simulink model "lookup_nD_TestGen18"  (R2017b)
settings: Solver=FixedStepDiscrete  StartTime=0.0  StopTime=10.0  RelTol=1e-3
model workspace (MAT data in the model file):
  LUTObjLKnD18 = Simulink.LookupTable
  LUTObjLKnD18.Table = Simulink.lookuptable.Table
  LUTObjLKnD18.Table.Value = reshape([4 16 10 5 19 18 6 20 23 7 21 24 8 22 25 4 16 10 5 19 18 6 20 23 7 21 24 8 22 25], [2 5 3])
  LUTObjLKnD18.Table.Dimensions = [2 5 3]
  LUTObjLKnD18.Table.DataType = 'auto'
  LUTObjLKnD18.Table.FieldName = 'Table'
  LUTObjLKnD18.BreakpointsSpecification = 'Even spacing'
  LUTObjLKnD18.Breakpoints(1) = Simulink.lookuptable.Evenspacing
  LUTObjLKnD18.Breakpoints(1).FirstPoint = 97.0345353457
  LUTObjLKnD18.Breakpoints(1).Spacing = 1.5
  LUTObjLKnD18.Breakpoints(1).FirstPointName = 'BPFirstPoint1'
  LUTObjLKnD18.Breakpoints(1).SpacingName = 'BPSpacing1'
  LUTObjLKnD18.Breakpoints(1).TunableSizeName = 'N1'
  LUTObjLKnD18.Breakpoints(1).DataType = 'auto'
  LUTObjLKnD18.Breakpoints(1).FieldName = 'BP1'
  LUTObjLKnD18.Breakpoints(2) = Simulink.lookuptable.Evenspacing
  LUTObjLKnD18.Breakpoints(2).FirstPoint = 71.1712484515
  LUTObjLKnD18.Breakpoints(2).Spacing = 1.5
  LUTObjLKnD18.Breakpoints(2).FirstPointName = 'BPFirstPoint2'
  LUTObjLKnD18.Breakpoints(2).SpacingName = 'BPSpacing2'
  LUTObjLKnD18.Breakpoints(2).TunableSizeName = 'N2'
  LUTObjLKnD18.Breakpoints(2).DataType = 'auto'
  LUTObjLKnD18.Breakpoints(2).FieldName = 'BP2'
  LUTObjLKnD18.Breakpoints(3) = Simulink.lookuptable.Evenspacing
  LUTObjLKnD18.Breakpoints(3).FirstPoint = 14.6088257293
  LUTObjLKnD18.Breakpoints(3).Spacing = 1.5
  LUTObjLKnD18.Breakpoints(3).FirstPointName = 'BPFirstPoint3'
  LUTObjLKnD18.Breakpoints(3).SpacingName = 'BPSpacing3'
  LUTObjLKnD18.Breakpoints(3).TunableSizeName = 'N3'
  LUTObjLKnD18.Breakpoints(3).DataType = 'auto'
  LUTObjLKnD18.Breakpoints(3).FieldName = 'BP3'
  LUTObjLKnD18.SupportTunableSize = 0
  LUTObjLKnD18.StructTypeInfo = Simulink.lookuptable.StructTypeInfo
  LUTObjLKnD18.StructTypeInfo.Name = 'LUT'
  LUTObjLKnD18.StructTypeInfo.DataScope = 'Auto'
settings Model: Creator=ktrinh  LastModifiedBy=ktrinh
settings DebuggingCC: ParameterOverflowMsg=none

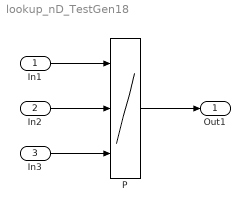
== system lookup_nD_TestGen18 ==
  In1 : Inport  OutMin=0  OutMax=127  PortDimensions=1
  In2 : Inport  Port=2  OutMin=0  OutMax=127
  In3 : Inport  Port=3  OutMin=0  OutMax=127
  P : Lookup_n-D  NumberOfTableDimensions=3  DataSpecification=Lookup table object  LookupTableObject=LUTObjLKnD18  BreakpointsSpecification=Even spacing  BreakpointsForDimension3=[5, 7]  Table=reshape(repmat([4 5 6;16 19 20;10 18 23],1,2),[3,3,2])  InternalRulePriority=Speed  RndMeth=Simplest  InputSameDT=on
  Out1 : Outport
  wires:
  In1/1 -> P/1
  In2/1 -> P/2
  In3/1 -> P/3
  P/1 -> Out1/1
